simulink library "cdsFiltMuxMatrix"  (Simulink 6.5)
settings Model: Creator=aivanov  LastModifiedBy=aivanov  ExtModeAutoUpdateStatusClock=off

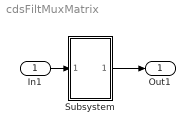
== system cdsFiltMuxMatrix ==
  In1 : Inport
  Subsystem : Subsystem
  Out1 : Outport
  wires:
  Subsystem/1(Out1) -> Out1/1
  In1/1 -> Subsystem/1(In1)

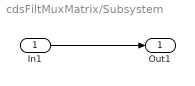
== system cdsFiltMuxMatrix/Subsystem ==
  In1 : Inport
  Out1 : Outport
  wires:
  In1/1 -> Out1/1
